simulink model "sampleModel106"  (R2022a)
settings: Solver=VariableStepAuto  StartTime=0.0  StopTime=10.0  RelTol=1e-3
undefined symbols (not defined in the file): DiscIntNeverNeededParam, magnitude, Newton, Raphson
libraries: simulink x379, slpidlib x89
(part 7 of 16)

== system sampleModel106/cfblk74/cfblk13/cfblk11/cfblk9 ==
  cfblk1 : Inport
  cfblk9 : Inport  Port=2
  cfblk10 : Inport  Port=3
  cfblk3 : slpidlib/PID Controller (2DOF)  Controller=PID  Form=Parallel  TimeDomain=Discrete-time  UseExternalTs=off  SampleTime=1  IntegratorMethod=Forward Euler  FilterMethod=Forward Euler  ControllerParametersSource=internal  P=1  I=1  UseKiTs=off  D=0  N=100  UseFilter=on  b=1  c=1  TunerSelectOption=Transfer Function Based (PID Tuner App)  InitialConditionSource=internal  InitialConditionForIntegrator=0  InitialConditionForFilter=0  DifferentiatorICPrevScaledInput=0  ExternalReset=none  TrackingMode=off  Kt=1  LimitOutput=off  SatLimitsSource=internal  UpperSaturationLimit=inf  LowerSaturationLimit=-inf  LinearizeAsGain=off  AntiWindupMode=none  Kb=1  POutMin=[]  POutMax=[]  IOutMin=[]  IOutMax=[]  DOutMin=[]  DOutMax=[]  NOutMin=[]  NOutMax=[]  bOutMin=[]  bOutMax=[]  cOutMin=[]  cOutMax=[]  SumOutMin=[]  SumOutMax=[]  SaturationOutMin=[]  SaturationOutMax=[]  PParamMin=[]  PParamMax=[]  IParamMin=[]  IParamMax=[]  DParamMin=[]  DParamMax=[]  NParamMin=[]  NParamMax=[]  bParamMin=[]  bParamMax=[]  cParamMin=[]  cParamMax=[]  KbParamMin=[]  KbParamMax=[]  KtParamMin=[]  KtParamMax=[]  KbOutMin=[]  KbOutMax=[]  KtOutMin=[]  KtOutMax=[]  IntegratorOutMin=[]  IntegratorOutMax=[]  FilterOutMin=[]  FilterOutMax=[]  SumI1OutMin=[]  SumI1OutMax=[]  SumI2OutMin=[]  SumI2OutMax=[]  SumI3OutMin=[]  SumI3OutMax=[]  SumI4OutMin=[]  SumI4OutMax=[]  SumDOutMin=[]  SumDOutMax=[]  Sum1OutMin=[]  Sum1OutMax=[]  Sum2OutMin=[]  Sum2OutMax=[]  Sum3OutMin=[]  Sum3OutMax=[]  DifferentiatorOutMin=[]  DifferentiatorOutMax=[]  FilterDiffOutCoefMin=[]  FilterDiffOutCoefMax=[]  ReciprocalOutMin=[]  ReciprocalOutMax=[]  SumDenOutMin=[]  SumDenOutMax=[]  SumNumOutMin=[]  SumNumOutMax=[]  DivideOutMin=[]  DivideOutMax=[]  UdiffTsProdOutMin=[]  UdiffTsProdOutMax=[]  NTsProdOutMin=[]  NTsProdOutMax=[]  UintegralTsProdOutMin=[]  UintegralTsProdOutMax=[]  UngainTsProdOutMin=[]  UngainTsProdOutMax=[]  IntegratorContinuousStateAttributes=''  IntegratorStateMustResolveToSignalObject=off  IntegratorRTWStateStorageClass=Auto  FilterContinuousStateAttributes=''  FilterStateMustResolveToSignalObject=off  FilterRTWStateStorageClass=Auto  ParallelPVariant=InternalParameters  IdealPVariant=Disabled  IVariant=InternalParameters  DVariant=InternalParameters  bVariant=InternalParameters  cVariant=InternalParameters  IntegratorVariant=Discrete  SatVariant=Disabled  AWVariant=Passthrough  PCopyVariant=Disabled  TRVariant=Disabled  FdbkBlocksVariant=Forward  IdealPFdbkVariant=Disabled  SatFdbkVariant=Disabled  DerivativeFilterVariant=ForwardEulerFilter  NVariant=InternalParameters  NCopyVariant=Disabled  FilterICVariant=InternalICsFilter  IntegratorICVariant=InternalICs  ExternalResetVariant=Disabled  TRSumVariant=Passthrough  SumFdbkVariant=Disabled  SumVariant=Sum_PID  TsampFilterVariant=InternalTs  TsampNgainVariant=Passthrough  TsampIntegralVariant=Passthrough  ExternalSaturationOutDataTypeStr=Inherit: Same as second input
      settings: SourceProductBaseCode=SL
  cfblk4 : simulink/Discrete/Difference  ICPrevInput=0.0  OutMin=[]  OutMax=[]  OutDataTypeStr=Inherit: Inherit via back propagation  OutDataType=fixdt(1, 16)  OutScaling=2^-10  DoSatur=off
  cfblk5 : Delay  SampleTime=1
  cfblk6 : Constant  Value=[-806684680.192649]  SampleTime=1
  cfblk7 : Constant  Value=[-623429069.453188]  SampleTime=1
  cfblk8 : Constant  Value=[-163983169.490583]  SampleTime=1
  cfblk2 : Outport
  cfblk11 : Outport  Port=2
  cfblk12 : Outport  Port=3
  wires:
  cfblk8/1 -> cfblk11/1
  cfblk6/1 -> cfblk2/1
  cfblk7/1 -> cfblk12/1
  cfblk10/1 -> cfblk5/1
  cfblk5/1 -> cfblk3/1
  cfblk9/1 -> cfblk3/2
  cfblk3/1 -> cfblk4/1

== system sampleModel106/cfblk74/cfblk13/cfblk12/cfblk10 ==
  cfblk1 : Inport
  cfblk8 : Inport  Port=2
  cfblk9 : Inport  Port=3
  cfblk3 : Delay  SampleTime=1
  cfblk4 : Sin  TimeSource=Use external signal  SampleTime=0
  cfblk5 : Sum  Inputs=+
  cfblk6 : simulink/Math Operations/MinMax Running Resettable  Function=min  vinit=0.0
  cfblk7 : Constant  Value=[-796301996.468178]  SampleTime=1
  cfblk2 : Outport
  cfblk10 : Outport  Port=2
  wires:
  cfblk5/1 -> cfblk4/1
  cfblk4/1 -> cfblk10/1
  cfblk8/1 -> cfblk6/1
  cfblk9/1 -> cfblk2/1
  cfblk3/1 -> cfblk5/1
  cfblk6/1 -> cfblk3/1
  cfblk7/1 -> cfblk6/2

== system sampleModel106/cfblk74/cfblk13/cfblk13/cfblk10 ==
  cfblk1 : Inport
  cfblk12 : Inport  Port=2
  cfblk13 : Inport  Port=3
  cfblk14 : Inport  Port=4
  cfblk15 : Inport  Port=5
  cfblk10 : ComplexToMagnitudeAngle
  cfblk11 : Constant  Value=[-793901753.508385]  SampleTime=1
  cfblk3 : simulink/Discrete/Transfer Fcn First Order  PoleZ=0.95  ICPrevOutput=0.0  DoSatur=off
  cfblk4 : MinMax  Inputs=3
  cfblk5 : Sum  Inputs=--
  cfblk6 : Rounding
  cfblk7 : UnaryMinus
  cfblk8 : Sqrt
  cfblk9 : Product
  cfblk2 : Outport
  cfblk16 : Outport  Port=2
  wires:
  cfblk7/1 -> cfblk5/1
  cfblk10/1 -> cfblk3/1
  cfblk10/2 -> cfblk7/1
  cfblk12/1 -> cfblk6/1
  cfblk6/1 -> cfblk10/1
  cfblk4/1 -> cfblk16/1
  cfblk11/1 -> cfblk5/2
  cfblk15/1 -> cfblk4/1
  cfblk3/1 -> cfblk8/1
  cfblk8/1 -> cfblk2/1
  cfblk5/1 -> cfblk9/1
  cfblk9/1 -> cfblk4/2
  cfblk14/1 -> cfblk4/3
  cfblk13/1 -> cfblk9/2

== system sampleModel106/cfblk74/cfblk13/cfblk13/cfblk11 ==
  cfblk1 : Inport
  cfblk3 : Product  Inputs=*
  cfblk4 : Sqrt
  cfblk5 : Bias  Bias=[715168761.956103]  SaturateOnIntegerOverflow=off
  cfblk6 : ComplexToMagnitudeAngle
  cfblk7 : Signum
  cfblk8 : Delay  SampleTime=1
  cfblk9 : Delay  SampleTime=1
  cfblk2 : Outport
  wires:
  cfblk1/1 -> cfblk2/1
  cfblk4/1 -> cfblk5/1
  cfblk3/1 -> cfblk7/1
  cfblk7/1 -> cfblk6/1
  cfblk6/1 -> cfblk8/1
  cfblk8/1 -> cfblk3/1
  cfblk5/1 -> cfblk9/1
  cfblk9/1 -> cfblk4/1

== system sampleModel106/cfblk74/cfblk13/cfblk13/cfblk12 ==
  cfblk1 : Inport
  cfblk10 : Constant  Value=[-475820294.361022]  SampleTime=1
  cfblk11 : Constant  Value=[-225279314.465098]  SampleTime=1
  cfblk3 : simulink/Discrete/Transfer Fcn Lead or Lag  PoleZ=0.95  ZeroZ=0.75  ICPrevOutput=0.0  ICPrevInput=0.0  DoSatur=off
      settings: SourceProductBaseCode=SL
  cfblk4 : Trigonometry
  cfblk5 : Sum  Inputs=|++
  cfblk6 : Squeeze
  cfblk7 : Reshape
  cfblk8 : Constant  Value=[-614077669.222538]  SampleTime=1
  cfblk9 : Constant  Value=[-535025394.973729]  SampleTime=1
  cfblk2 : Outport
  cfblk12 : Outport  Port=2
  wires:
  cfblk5/1 -> cfblk3/1
  cfblk11/1 -> cfblk12/1
  cfblk8/1 -> cfblk7/1
  cfblk4/1 -> cfblk2/1
  cfblk9/1 -> cfblk4/1
  cfblk3/1 -> cfblk6/1
  cfblk1/1 -> cfblk5/1
  cfblk7/1 -> cfblk5/2

== system sampleModel106/cfblk74/cfblk13/cfblk13/cfblk9 ==
  cfblk1 : Inport
  cfblk7 : Inport  Port=2
  cfblk3 : simulink/Discrete/Transfer Fcn Real Zero  ZeroZ=0.75  ICPrevInput=0.0  DoSatur=off
      settings: SourceProductBaseCode=SL
  cfblk4 : Reshape
  cfblk5 : Rounding
  cfblk6 : Constant  Value=[-810853108.486231]  SampleTime=1
  cfblk2 : Outport
  cfblk8 : Outport  Port=2
  wires:
  cfblk4/1 -> cfblk3/1
  cfblk1/1 -> cfblk2/1
  cfblk7/1 -> cfblk5/1
  cfblk6/1 -> cfblk4/1
  cfblk5/1 -> cfblk8/1

== system sampleModel106/cfblk74/cfblk9/cfblk11/cfblk8 ==
  cfblk1 : Inport
  cfblk9 : Inport  Port=2
  cfblk10 : Inport  Port=3
  cfblk3 : Delay  ShowEnablePort=on  SampleTime=1
      settings: InputPortMap=u0,e6
  cfblk4 : Sqrt  Operator=rSqrt  AlgorithmType=Newton-Raphson
  cfblk5 : simulink/Math Operations/MinMax Running Resettable  Function=min  vinit=0.0
  cfblk6 : Constant  Value=[-597140278.382424]  SampleTime=1
  cfblk7 : Constant  Value=[926673631.119186]  SampleTime=1
  cfblk8 : Constant  Value=[-242832753.012015]  SampleTime=1
  cfblk2 : Outport
  cfblk11 : Outport  Port=2
  wires:
  cfblk10/1 -> cfblk11/1
  cfblk4/1 -> cfblk3/1
  cfblk9/1 -> cfblk5/1
  cfblk5/1 -> cfblk2/1
  cfblk8/1 -> cfblk3/2
  cfblk6/1 -> cfblk5/2
  cfblk1/1 -> cfblk4/1

== system sampleModel106/cfblk74/cfblk9/cfblk11/cfblk9 ==
  cfblk1 : Inport
  cfblk8 : Inport  Port=2
  cfblk3 : Signum
  cfblk4 : Sum  Inputs=+-
  cfblk5 : PermuteDimensions
  cfblk6 : Product  Inputs=**
  cfblk7 : Constant  Value=[458452339.303576]  SampleTime=1
  cfblk2 : Outport
  cfblk9 : Outport  Port=2
  wires:
  cfblk5/1 -> cfblk6/1
  cfblk7/1 -> cfblk4/1
  cfblk3/1 -> cfblk6/2
  cfblk6/1 -> cfblk9/1
  cfblk8/1 -> cfblk4/2, cfblk5/1
  cfblk1/1 -> cfblk2/1
  cfblk4/1 -> cfblk3/1

== system sampleModel106/cfblk74/cfblk9/cfblk12/cfblk10 ==
  cfblk1 : Inport
  cfblk6 : Inport  Port=2
  cfblk7 : Inport  Port=3
  cfblk3 : slpidlib/PID Controller (2DOF)  Controller=PID  Form=Parallel  TimeDomain=Discrete-time  UseExternalTs=off  SampleTime=1  IntegratorMethod=Forward Euler  FilterMethod=Forward Euler  ControllerParametersSource=internal  P=1  I=1  UseKiTs=off  D=0  N=100  UseFilter=on  b=1  c=1  TunerSelectOption=Transfer Function Based (PID Tuner App)  InitialConditionSource=internal  InitialConditionForIntegrator=0  InitialConditionForFilter=0  DifferentiatorICPrevScaledInput=0  ExternalReset=none  TrackingMode=off  Kt=1  LimitOutput=off  SatLimitsSource=internal  UpperSaturationLimit=inf  LowerSaturationLimit=-inf  LinearizeAsGain=off  AntiWindupMode=none  Kb=1  POutMin=[]  POutMax=[]  IOutMin=[]  IOutMax=[]  DOutMin=[]  DOutMax=[]  NOutMin=[]  NOutMax=[]  bOutMin=[]  bOutMax=[]  cOutMin=[]  cOutMax=[]  SumOutMin=[]  SumOutMax=[]  SaturationOutMin=[]  SaturationOutMax=[]  PParamMin=[]  PParamMax=[]  IParamMin=[]  IParamMax=[]  DParamMin=[]  DParamMax=[]  NParamMin=[]  NParamMax=[]  bParamMin=[]  bParamMax=[]  cParamMin=[]  cParamMax=[]  KbParamMin=[]  KbParamMax=[]  KtParamMin=[]  KtParamMax=[]  KbOutMin=[]  KbOutMax=[]  KtOutMin=[]  KtOutMax=[]  IntegratorOutMin=[]  IntegratorOutMax=[]  FilterOutMin=[]  FilterOutMax=[]  SumI1OutMin=[]  SumI1OutMax=[]  SumI2OutMin=[]  SumI2OutMax=[]  SumI3OutMin=[]  SumI3OutMax=[]  SumI4OutMin=[]  SumI4OutMax=[]  SumDOutMin=[]  SumDOutMax=[]  Sum1OutMin=[]  Sum1OutMax=[]  Sum2OutMin=[]  Sum2OutMax=[]  Sum3OutMin=[]  Sum3OutMax=[]  DifferentiatorOutMin=[]  DifferentiatorOutMax=[]  FilterDiffOutCoefMin=[]  FilterDiffOutCoefMax=[]  ReciprocalOutMin=[]  ReciprocalOutMax=[]  SumDenOutMin=[]  SumDenOutMax=[]  SumNumOutMin=[]  SumNumOutMax=[]  DivideOutMin=[]  DivideOutMax=[]  UdiffTsProdOutMin=[]  UdiffTsProdOutMax=[]  NTsProdOutMin=[]  NTsProdOutMax=[]  UintegralTsProdOutMin=[]  UintegralTsProdOutMax=[]  UngainTsProdOutMin=[]  UngainTsProdOutMax=[]  IntegratorContinuousStateAttributes=''  IntegratorStateMustResolveToSignalObject=off  IntegratorRTWStateStorageClass=Auto  FilterContinuousStateAttributes=''  FilterStateMustResolveToSignalObject=off  FilterRTWStateStorageClass=Auto  ParallelPVariant=InternalParameters  IdealPVariant=Disabled  IVariant=InternalParameters  DVariant=InternalParameters  bVariant=InternalParameters  cVariant=InternalParameters  IntegratorVariant=Discrete  SatVariant=Disabled  AWVariant=Passthrough  PCopyVariant=Disabled  TRVariant=Disabled  FdbkBlocksVariant=Forward  IdealPFdbkVariant=Disabled  SatFdbkVariant=Disabled  DerivativeFilterVariant=ForwardEulerFilter  NVariant=InternalParameters  NCopyVariant=Disabled  FilterICVariant=InternalICsFilter  IntegratorICVariant=InternalICs  ExternalResetVariant=Disabled  TRSumVariant=Passthrough  SumFdbkVariant=Disabled  SumVariant=Sum_PID  TsampFilterVariant=InternalTs  TsampNgainVariant=Passthrough  TsampIntegralVariant=Passthrough  ExternalSaturationOutDataTypeStr=Inherit: Same as second input
      settings: SourceProductBaseCode=SL
  cfblk4 : DiscreteZeroPole  Poles=[0 0.5]  Gain=1
  cfblk5 : Gain  Gain=[955284268.719632]
  cfblk8 : Delay  SampleTime=1
  cfblk2 : Outport
  wires:
  cfblk5/1 -> cfblk4/1
  cfblk1/1 -> cfblk3/1
  cfblk3/1 -> cfblk5/1
  cfblk6/1 -> cfblk2/1
  cfblk4/1 -> cfblk8/1
  cfblk8/1 -> cfblk3/2

== system sampleModel106/cfblk74/cfblk9/cfblk12/cfblk13 ==
  cfblk1 : Inport
  cfblk12 : Inport  Port=2
  cfblk13 : Inport  Port=3
  Action Port : ActionPort  ActionPortLabel=if(u1 >= 0)
  cfblk10 : Constant  Value=[-679946503.878796]  SampleTime=1
  cfblk11 : Constant  Value=[-962530128.203573]  SampleTime=1
  cfblk17 : Delay
  cfblk3 : Sum
  cfblk4 : Sum  Inputs=+-
  cfblk5 : Trigonometry
  cfblk6 : Sum  Inputs=+-
  cfblk7 : Squeeze
  cfblk8 : Constant  Value=[916836463.739358]  SampleTime=1
  cfblk9 : Constant  Value=[-400818000.791556]  SampleTime=1
  cfblk2 : Outport
  cfblk14 : Outport  Port=2
  cfblk15 : Outport  Port=3
  cfblk16 : Outport  Port=4
  wires:
  cfblk3/1 -> cfblk4/1
  cfblk11/1 -> cfblk14/1
  cfblk5/1 -> cfblk2/1
  cfblk7/1 -> cfblk3/1
  cfblk9/1 -> cfblk15/1
  cfblk12/1 -> cfblk6/1
  cfblk6/1 -> cfblk4/2
  cfblk1/1 -> cfblk16/1
  cfblk8/1 -> cfblk7/1
  cfblk13/1 -> cfblk6/2
  cfblk10/1 -> cfblk5/1
  cfblk4/1 -> cfblk17/1
  cfblk17/1 -> cfblk3/2

== system sampleModel106/cfblk74/cfblk9/cfblk12/cfblk14 ==
  cfblk1 : Inport
  cfblk9 : Inport  Port=2
  cfblk10 : Inport  Port=3
  cfblk11 : Inport  Port=4
  Action Port : ActionPort  ActionPortLabel=else
  cfblk3 : DiscreteTransferFcn
  cfblk4 : Squeeze
  cfblk5 : Product
  cfblk6 : Constant  Value=[-850030709.629340]  SampleTime=1
  cfblk7 : Constant  Value=[320075082.603753]  SampleTime=1
  cfblk8 : Constant  Value=[416679782.582926]  SampleTime=1
  cfblk2 : Outport
  cfblk12 : Outport  Port=2
  wires:
  cfblk6/1 -> cfblk5/1
  cfblk11/1 -> cfblk4/1
  cfblk5/1 -> cfblk2/1
  cfblk4/1 -> cfblk3/1
  cfblk1/1 -> cfblk5/2
  cfblk3/1 -> cfblk12/1

== system sampleModel106/cfblk74/cfblk9/cfblk12/cfblk8 ==
  cfblk1 : Inport
  cfblk7 : Inport  Port=2
  cfblk3 : PermuteDimensions
  cfblk4 : simulink/Math Operations/Slider Gain  gain=1  low=0  high=2
  cfblk5 : Gain  Gain=[356985907.848455]
  cfblk6 : Sum  Inputs=+-
  cfblk8 : Delay  SampleTime=1
  cfblk2 : Outport
  wires:
  cfblk7/1 -> cfblk2/1, cfblk5/1
  cfblk6/1 -> cfblk4/1
  cfblk1/1 -> cfblk3/1
  cfblk3/1 -> cfblk6/2
  cfblk4/1 -> cfblk8/1
  cfblk8/1 -> cfblk6/1

== system sampleModel106/cfblk74/cfblk9/cfblk12/cfblk9 ==
  cfblk1 : Inport
  cfblk8 : Inport  Port=2
  cfblk9 : Inport  Port=3
  cfblk10 : Inport  Port=4
  cfblk3 : simulink/Discrete/Transfer Fcn Lead or Lag  PoleZ=0.95  ZeroZ=0.75  ICPrevOutput=0.0  ICPrevInput=0.0  DoSatur=off
      settings: SourceProductBaseCode=SL
  cfblk4 : ComplexToMagnitudeAngle
  cfblk5 : Rounding
  cfblk6 : Sum  Inputs=-+
  cfblk7 : Gain  Gain=[630253926.006221]
  cfblk2 : Outport
  wires:
  cfblk6/1 -> cfblk5/1
  cfblk3/1 -> cfblk7/1
  cfblk10/1 -> cfblk6/1
  cfblk5/1 -> cfblk4/1
  cfblk1/1 -> cfblk6/2
  cfblk8/1 -> cfblk2/1
  cfblk9/1 -> cfblk3/1

== system sampleModel106/cfblk74/cfblk9/cfblk13/cfblk5 ==
  cfblk1 : Inport
  cfblk9 : Inport  Port=2
  cfblk3 : DiscreteFir  SampleTime=1
  cfblk4 : DiscreteIntegrator  ICPrevOutput=DiscIntNeverNeededParam  ICPrevScaledInput=DiscIntNeverNeededParam
  cfblk5 : slpidlib/PID Controller  Controller=PID  Form=Parallel  TimeDomain=Discrete-time  UseExternalTs=off  SampleTime=1  IntegratorMethod=Forward Euler  FilterMethod=Forward Euler  ControllerParametersSource=internal  P=1  I=1  UseKiTs=off  D=0  N=100  UseFilter=on  TunerSelectOption=Transfer Function Based (PID Tuner App)  InitialConditionSource=internal  InitialConditionForIntegrator=0  InitialConditionForFilter=0  DifferentiatorICPrevScaledInput=0  ExternalReset=none  TrackingMode=off  Kt=1  LimitOutput=off  SatLimitsSource=internal  UpperSaturationLimit=inf  LowerSaturationLimit=-inf  LinearizeAsGain=off  AntiWindupMode=none  Kb=1  POutMin=[]  POutMax=[]  IOutMin=[]  IOutMax=[]  DOutMin=[]  DOutMax=[]  NOutMin=[]  NOutMax=[]  SumOutMin=[]  SumOutMax=[]  SaturationOutMin=[]  SaturationOutMax=[]  PParamMin=[]  PParamMax=[]  IParamMin=[]  IParamMax=[]  DParamMin=[]  DParamMax=[]  NParamMin=[]  NParamMax=[]  KbParamMin=[]  KbParamMax=[]  KtParamMin=[]  KtParamMax=[]  KbOutMin=[]  KbOutMax=[]  KtOutMin=[]  KtOutMax=[]  IntegratorOutMin=[]  IntegratorOutMax=[]  FilterOutMin=[]  FilterOutMax=[]  SumI1OutMin=[]  SumI1OutMax=[]  SumI2OutMin=[]  SumI2OutMax=[]  SumI3OutMin=[]  SumI3OutMax=[]  SumI4OutMin=[]  SumI4OutMax=[]  SumDOutMin=[]  SumDOutMax=[]  DifferentiatorOutMin=[]  DifferentiatorOutMax=[]  FilterDiffOutCoefMin=[]  FilterDiffOutCoefMax=[]  ReciprocalOutMin=[]  ReciprocalOutMax=[]  SumDenOutMin=[]  SumDenOutMax=[]  SumNumOutMin=[]  SumNumOutMax=[]  DivideOutMin=[]  DivideOutMax=[]  UdiffTsProdOutMin=[]  UdiffTsProdOutMax=[]  NTsProdOutMin=[]  NTsProdOutMax=[]  UintegralTsProdOutMin=[]  UintegralTsProdOutMax=[]  UngainTsProdOutMin=[]  UngainTsProdOutMax=[]  IntegratorContinuousStateAttributes=''  IntegratorStateMustResolveToSignalObject=off  IntegratorRTWStateStorageClass=Auto  FilterContinuousStateAttributes=''  FilterStateMustResolveToSignalObject=off  FilterRTWStateStorageClass=Auto  ParallelPVariant=InternalParameters  IdealPVariant=Disabled  IVariant=InternalParameters  DVariant=InternalParameters  IntegratorVariant=Discrete  SatVariant=Disabled  AWVariant=Passthrough  PCopyVariant=Disabled  TRVariant=Disabled  FdbkBlocksVariant=Forward  IdealPFdbkVariant=Disabled  SatFdbkVariant=Disabled  DerivativeFilterVariant=ForwardEulerFilter  NVariant=InternalParameters  NCopyVariant=Disabled  FilterICVariant=InternalICsFilter  IntegratorICVariant=InternalICs  ExternalResetVariant=Disabled  TRSumVariant=Passthrough  SumFdbkVariant=Disabled  SumVariant=Sum_PID  TsampFilterVariant=InternalTs  TsampNgainVariant=Passthrough  TsampIntegralVariant=Passthrough  ExternalSaturationOutDataTypeStr=Inherit: Same as second input  aMode=0
  cfblk6 : MinMax
  cfblk7 : Gain  Gain=[65666299.408699]
  cfblk8 : Constant  Value=[554029224.863969]  SampleTime=1
  cfblk2 : Outport
  cfblk10 : Outport  Port=2
  wires:
  cfblk6/1 -> cfblk5/1
  cfblk8/1 -> cfblk7/1
  cfblk9/1 -> cfblk10/1
  cfblk7/1 -> cfblk6/1
  cfblk5/1 -> cfblk3/1
  cfblk3/1 -> cfblk4/1
  cfblk1/1 -> cfblk2/1

== system sampleModel106/cfblk74/cfblk9/cfblk13/cfblk6 ==
  cfblk1 : Inport
  cfblk7 : Inport  Port=2
  cfblk8 : Inport  Port=3
  cfblk10 : Delay  SampleTime=1
  cfblk3 : DiscreteTransferFcn  SampleTime=1
  cfblk4 : UnitDelay  HasFrameUpgradeWarning=on
  cfblk5 : DiscreteIntegrator  ICPrevOutput=DiscIntNeverNeededParam  ICPrevScaledInput=DiscIntNeverNeededParam
  cfblk6 : UnaryMinus
  cfblk2 : Outport
  cfblk9 : Outport  Port=2
  wires:
  cfblk5/1 -> cfblk2/1
  cfblk3/1 -> cfblk4/1
  cfblk1/1 -> cfblk9/1
  cfblk4/1 -> cfblk6/1
  cfblk7/1 -> cfblk5/1
  cfblk6/1 -> cfblk10/1
  cfblk10/1 -> cfblk3/1

== system sampleModel106/cfblk74/cfblk9/cfblk13/cfblk7 ==
  cfblk1 : Inport
  cfblk10 : Sqrt
  cfblk11 : Constant  Value=[49726155.340751]  SampleTime=1
  cfblk12 : Constant  Value=[51502285.530327]  SampleTime=1
  cfblk14 : Delay  SampleTime=1
  cfblk3 : simulink/Discrete/Transfer Fcn Lead or Lag  PoleZ=0.95  ZeroZ=0.75  ICPrevOutput=0.0  ICPrevInput=0.0  DoSatur=off
      settings: SourceProductBaseCode=SL
  cfblk4 : Sum  Inputs=+-
  cfblk5 : Trigonometry
  cfblk6 : simulink/Math Operations/Slider Gain  gain=1  low=0  high=2
  cfblk7 : MinMax  Function=max  Inputs=2
  cfblk8 : Sqrt
  cfblk9 : Math  Operator=10^u
  cfblk2 : Outport
  cfblk13 : Outport  Port=2
  wires:
  cfblk1/1 -> cfblk5/1
  cfblk12/1 -> cfblk3/1
  cfblk4/1 -> cfblk8/1
  cfblk9/1 -> cfblk6/1
  cfblk3/1 -> cfblk9/1, cfblk4/2
  cfblk6/1 -> cfblk2/1
  cfblk8/1 -> cfblk10/1
  cfblk5/1 -> cfblk7/1
  cfblk11/1 -> cfblk7/2
  cfblk7/1 -> cfblk13/1
  cfblk10/1 -> cfblk14/1
  cfblk14/1 -> cfblk4/1

== system sampleModel106/cfblk74/cfblk9/cfblk15/cfblk10 ==
  cfblk1 : Inport
  cfblk11 : Inport  Port=2
  cfblk10 : Constant  Value=[231958979.755721]  SampleTime=1
  cfblk3 : DiscreteFilter  SampleTime=1
  cfblk4 : Product  Inputs=*
  cfblk5 : Gain  Gain=[-64902621.159940]
  cfblk6 : Reshape
  cfblk7 : Sum  Inputs=+
  cfblk8 : Constant  Value=[-549811752.008296]  SampleTime=1
  cfblk9 : Constant  Value=[666189529.416412]  SampleTime=1
  cfblk2 : Outport
  cfblk12 : Outport  Port=2
  wires:
  cfblk9/1 -> cfblk6/1
  cfblk1/1 -> cfblk3/1
  cfblk6/1 -> cfblk5/1
  cfblk10/1 -> cfblk7/1
  cfblk5/1 -> cfblk2/1
  cfblk11/1 -> cfblk4/1
  cfblk3/1 -> cfblk12/1

== system sampleModel106/cfblk74/cfblk9/cfblk15/cfblk11 ==
  cfblk1 : Inport
  cfblk13 : Inport  Port=2
  cfblk14 : Inport  Port=3
  cfblk10 : Constant  Value=[-458676472.570737]  SampleTime=1
  cfblk11 : Constant  Value=[-707014969.582165]  SampleTime=1
  cfblk12 : Constant  Value=[815086080.140174]  SampleTime=1
  cfblk17 : Delay  SampleTime=1
  cfblk3 : slpidlib/PID Controller (2DOF)  Controller=PID  Form=Parallel  TimeDomain=Discrete-time  UseExternalTs=off  SampleTime=1  IntegratorMethod=Forward Euler  FilterMethod=Forward Euler  ControllerParametersSource=internal  P=1  I=1  UseKiTs=off  D=0  N=100  UseFilter=on  b=1  c=1  TunerSelectOption=Transfer Function Based (PID Tuner App)  InitialConditionSource=internal  InitialConditionForIntegrator=0  InitialConditionForFilter=0  DifferentiatorICPrevScaledInput=0  ExternalReset=none  TrackingMode=off  Kt=1  LimitOutput=off  SatLimitsSource=internal  UpperSaturationLimit=inf  LowerSaturationLimit=-inf  LinearizeAsGain=off  AntiWindupMode=none  Kb=1  POutMin=[]  POutMax=[]  IOutMin=[]  IOutMax=[]  DOutMin=[]  DOutMax=[]  NOutMin=[]  NOutMax=[]  bOutMin=[]  bOutMax=[]  cOutMin=[]  cOutMax=[]  SumOutMin=[]  SumOutMax=[]  SaturationOutMin=[]  SaturationOutMax=[]  PParamMin=[]  PParamMax=[]  IParamMin=[]  IParamMax=[]  DParamMin=[]  DParamMax=[]  NParamMin=[]  NParamMax=[]  bParamMin=[]  bParamMax=[]  cParamMin=[]  cParamMax=[]  KbParamMin=[]  KbParamMax=[]  KtParamMin=[]  KtParamMax=[]  KbOutMin=[]  KbOutMax=[]  KtOutMin=[]  KtOutMax=[]  IntegratorOutMin=[]  IntegratorOutMax=[]  FilterOutMin=[]  FilterOutMax=[]  SumI1OutMin=[]  SumI1OutMax=[]  SumI2OutMin=[]  SumI2OutMax=[]  SumI3OutMin=[]  SumI3OutMax=[]  SumI4OutMin=[]  SumI4OutMax=[]  SumDOutMin=[]  SumDOutMax=[]  Sum1OutMin=[]  Sum1OutMax=[]  Sum2OutMin=[]  Sum2OutMax=[]  Sum3OutMin=[]  Sum3OutMax=[]  DifferentiatorOutMin=[]  DifferentiatorOutMax=[]  FilterDiffOutCoefMin=[]  FilterDiffOutCoefMax=[]  ReciprocalOutMin=[]  ReciprocalOutMax=[]  SumDenOutMin=[]  SumDenOutMax=[]  SumNumOutMin=[]  SumNumOutMax=[]  DivideOutMin=[]  DivideOutMax=[]  UdiffTsProdOutMin=[]  UdiffTsProdOutMax=[]  NTsProdOutMin=[]  NTsProdOutMax=[]  UintegralTsProdOutMin=[]  UintegralTsProdOutMax=[]  UngainTsProdOutMin=[]  UngainTsProdOutMax=[]  IntegratorContinuousStateAttributes=''  IntegratorStateMustResolveToSignalObject=off  IntegratorRTWStateStorageClass=Auto  FilterContinuousStateAttributes=''  FilterStateMustResolveToSignalObject=off  FilterRTWStateStorageClass=Auto  ParallelPVariant=InternalParameters  IdealPVariant=Disabled  IVariant=InternalParameters  DVariant=InternalParameters  bVariant=InternalParameters  cVariant=InternalParameters  IntegratorVariant=Discrete  SatVariant=Disabled  AWVariant=Passthrough  PCopyVariant=Disabled  TRVariant=Disabled  FdbkBlocksVariant=Forward  IdealPFdbkVariant=Disabled  SatFdbkVariant=Disabled  DerivativeFilterVariant=ForwardEulerFilter  NVariant=InternalParameters  NCopyVariant=Disabled  FilterICVariant=InternalICsFilter  IntegratorICVariant=InternalICs  ExternalResetVariant=Disabled  TRSumVariant=Passthrough  SumFdbkVariant=Disabled  SumVariant=Sum_PID  TsampFilterVariant=InternalTs  TsampNgainVariant=Passthrough  TsampIntegralVariant=Passthrough  ExternalSaturationOutDataTypeStr=Inherit: Same as second input
      settings: SourceProductBaseCode=SL
  cfblk4 : DiscreteTransferFcn  SampleTime=1
  cfblk5 : Delay  SampleTime=1
  cfblk6 : DiscreteIntegrator  ICPrevOutput=DiscIntNeverNeededParam  ICPrevScaledInput=DiscIntNeverNeededParam
  cfblk7 : Reshape
  cfblk8 : Squeeze
  cfblk9 : Constant  Value=[869825865.592683]  SampleTime=1
  cfblk2 : Outport
  cfblk15 : Outport  Port=2
  cfblk16 : Outport  Port=3
  wires:
  cfblk9/1 -> cfblk2/1
  cfblk10/1 -> cfblk6/1
  cfblk7/1 -> cfblk8/1
  cfblk5/1 -> cfblk16/1
  cfblk3/1 -> cfblk7/1
  cfblk13/1 -> cfblk5/1
  cfblk12/1 -> cfblk15/1
  cfblk1/1 -> cfblk4/1
  cfblk6/1 -> cfblk3/2
  cfblk8/1 -> cfblk17/1
  cfblk17/1 -> cfblk3/1

== system sampleModel106/cfblk74/cfblk9/cfblk15/cfblk9 ==
  cfblk1 : Inport
  cfblk7 : Inport  Port=2
  cfblk8 : Inport  Port=3
  cfblk3 : Delay  DelayLengthSource=Input port  SampleTime=1
      settings: InputPortMap=u0,p1
  cfblk4 : simulink/Discrete/Difference  ICPrevInput=0.0  OutMin=[]  OutMax=[]  OutDataTypeStr=Inherit: Inherit via back propagation  OutDataType=fixdt(1, 16)  OutScaling=2^-10  DoSatur=off
  cfblk5 : Product  Inputs=**
  cfblk6 : Constant  Value=[-105116644.466995]  SampleTime=1
  cfblk9 : Delay  SampleTime=1
  cfblk2 : Outport
  wires:
  cfblk6/1 -> cfblk3/1
  cfblk1/1 -> cfblk2/1
  cfblk4/1 -> cfblk5/1
  cfblk3/1 -> cfblk4/1
  cfblk8/1 -> cfblk5/2
  cfblk5/1 -> cfblk9/1
  cfblk9/1 -> cfblk3/2

== system sampleModel106/cfblk74/cfblk9/cfblk16/cfblk7 ==
  cfblk1 : Inport
  cfblk7 : Inport  Port=2
  cfblk8 : Inport  Port=3
  cfblk3 : simulink/Discrete/Difference  ICPrevInput=0.0  OutMin=[]  OutMax=[]  OutDataTypeStr=Inherit: Inherit via back propagation  OutDataType=fixdt(1, 16)  OutScaling=2^-10  DoSatur=off
  cfblk4 : ComplexToRealImag
  cfblk5 : Sum  Inputs=+-
  cfblk6 : Constant  Value=[101423658.427814]  SampleTime=1
  cfblk2 : Outport
  wires:
  cfblk4/1 -> cfblk5/1
  cfblk8/1 -> cfblk2/1
  cfblk7/1 -> cfblk4/1
  cfblk6/1 -> cfblk3/1
  cfblk3/1 -> cfblk5/2

== system sampleModel106/cfblk74/cfblk9/cfblk16/cfblk8 ==
  cfblk1 : Inport
  cfblk14 : Inport  Port=2
  cfblk15 : Inport  Port=3
  cfblk10 : Squeeze
  cfblk11 : Reshape
  cfblk12 : simulink/Math Operations/Slider Gain  gain=1  low=0  high=2
  cfblk13 : Constant  Value=[-734947851.856283]  SampleTime=1
  cfblk17 : Delay  SampleTime=1
  cfblk18 : Delay  SampleTime=1
  cfblk3 : Delay  ShowEnablePort=on  SampleTime=1
      settings: InputPortMap=u0,e6
  cfblk4 : Delay  SampleTime=1
  cfblk5 : DiscreteFilter  SampleTime=1
  cfblk6 : simulink/Discrete/Difference  ICPrevInput=0.0  OutMin=[]  OutMax=[]  OutDataTypeStr=Inherit: Inherit via back propagation  OutDataType=fixdt(1, 16)  OutScaling=2^-10  DoSatur=off
  cfblk7 : Trigonometry
  cfblk8 : MinMax  Function=max
  cfblk9 : Trigonometry
  cfblk2 : Outport
  cfblk16 : Outport  Port=2
  wires:
  cfblk12/1 -> cfblk10/1
  cfblk10/1 -> cfblk6/1
  cfblk14/1 -> cfblk2/1
  cfblk7/1 -> cfblk9/1
  cfblk15/1 -> cfblk16/1
  cfblk1/1 -> cfblk12/1
  cfblk11/1 -> cfblk8/1
  cfblk3/1 -> cfblk11/1
  cfblk13/1 -> cfblk4/1
  cfblk5/1 -> cfblk7/1
  cfblk6/1 -> cfblk3/1
  cfblk8/1 -> cfblk17/1
  cfblk17/1 -> cfblk3/2
  cfblk9/1 -> cfblk18/1
  cfblk18/1 -> cfblk5/1

== system sampleModel106/cfblk74/cfblk9/cfblk9/cfblk10 ==
  cfblk1 : Inport
  cfblk10 : Inport  Port=2
  cfblk11 : Inport  Port=3
  cfblk12 : Inport  Port=4
  cfblk13 : Delay  SampleTime=1
  cfblk3 : Delay  ShowEnablePort=on  SampleTime=1
      settings: InputPortMap=u0,e6
  cfblk4 : DiscreteStateSpace
  cfblk5 : Rounding
  cfblk6 : Abs  SaturateOnIntegerOverflow=off
  cfblk7 : Product  Inputs=*
  cfblk8 : Sum  Inputs=+-
  cfblk9 : Constant  Value=[839535444.416101]  SampleTime=1
  cfblk2 : Outport
  wires:
  cfblk3/1 -> cfblk4/1
  cfblk4/1 -> cfblk2/1
  cfblk11/1 -> cfblk8/1
  cfblk5/1 -> cfblk7/1
  cfblk9/1 -> cfblk3/1
  cfblk1/1 -> cfblk8/2
  cfblk12/1 -> cfblk6/1
  cfblk10/1 -> cfblk3/2
  cfblk7/1 -> cfblk13/1
  cfblk13/1 -> cfblk5/1

== system sampleModel106/cfblk74/cfblk9/cfblk9/cfblk11 ==
  cfblk1 : Inport
  cfblk6 : Inport  Port=2
  cfblk7 : Inport  Port=3
  cfblk8 : Inport  Port=4
  cfblk3 : Delay  ShowEnablePort=on  SampleTime=1
      settings: InputPortMap=u0,e6
  cfblk4 : simulink/Discrete/Transfer Fcn Lead or Lag  PoleZ=0.95  ZeroZ=0.75  ICPrevOutput=0.0  ICPrevInput=0.0  DoSatur=off
      settings: SourceProductBaseCode=SL
  cfblk5 : Sum  Inputs=|++
  cfblk9 : Delay  SampleTime=1
  cfblk2 : Outport
  wires:
  cfblk7/1 -> cfblk2/1
  cfblk1/1 -> cfblk3/1
  cfblk4/1 -> cfblk5/1
  cfblk6/1 -> cfblk3/2
  cfblk8/1 -> cfblk5/2
  cfblk5/1 -> cfblk9/1
  cfblk9/1 -> cfblk4/1

== system sampleModel106/cfblk74/cfblk9/cfblk9/cfblk9 ==
  cfblk1 : Inport
  cfblk10 : Constant  Value=[-213956286.197865]  SampleTime=1
  cfblk12 : Delay  SampleTime=1
  cfblk3 : DiscreteIntegrator  ICPrevOutput=DiscIntNeverNeededParam  ICPrevScaledInput=DiscIntNeverNeededParam
  cfblk4 : simulink/Math Operations/Slider Gain  gain=1  low=0  high=2
  cfblk5 : Gain  Gain=[-650980414.519220]
  cfblk6 : Sum
  cfblk7 : Bias  Bias=[254600432.308890]  SaturateOnIntegerOverflow=off
  cfblk8 : Sum
  cfblk9 : Constant  Value=[-488733431.313732]  SampleTime=1
  cfblk2 : Outport
  cfblk11 : Outport  Port=2
  wires:
  cfblk4/1 -> cfblk8/1
  cfblk9/1 -> cfblk11/1
  cfblk6/1 -> cfblk5/1
  cfblk5/1 -> cfblk2/1, cfblk12/1
  cfblk8/1 -> cfblk6/2
  cfblk10/1 -> cfblk3/1
  cfblk1/1 -> cfblk7/1
  cfblk3/1 -> cfblk8/2
  cfblk7/1 -> cfblk4/1
  cfblk12/1 -> cfblk6/1

== system sampleModel106/cfblk75/cfblk5/cfblk10/cfblk10 ==
  cfblk1 : Inport
  cfblk7 : Inport  Port=2
  Action Port : ActionPort  ActionPortLabel=if(u1 >= 0)
  cfblk3 : DiscreteFir
  cfblk4 : Sqrt  Operator=rSqrt  AlgorithmType=Newton-Raphson
  cfblk5 : ComplexToRealImag
  cfblk6 : Constant  Value=[-367349926.183283]  SampleTime=1
  cfblk2 : Outport
  wires:
  cfblk7/1 -> cfblk3/1
  cfblk1/1 -> cfblk5/1
  cfblk3/1 -> cfblk4/1
  cfblk4/1 -> cfblk2/1

== system sampleModel106/cfblk75/cfblk5/cfblk10/cfblk11 ==
  cfblk1 : Inport
  cfblk6 : Inport  Port=2
  cfblk7 : Inport  Port=3
  Action Port : ActionPort  ActionPortLabel=else
  cfblk3 : simulink/Discrete/Difference  ICPrevInput=0.0  OutMin=[]  OutMax=[]  OutDataTypeStr=Inherit: Inherit via back propagation  OutDataType=fixdt(1, 16)  OutScaling=2^-10  DoSatur=off
  cfblk4 : Rounding
  cfblk5 : UnaryMinus
  cfblk2 : Outport
  wires:
  cfblk1/1 -> cfblk4/1
  cfblk7/1 -> cfblk3/1
  cfblk6/1 -> cfblk5/1
  cfblk3/1 -> cfblk2/1

== system sampleModel106/cfblk75/cfblk5/cfblk10/cfblk7 ==
  cfblk1 : Inport
  cfblk8 : Inport  Port=2
  cfblk9 : Inport  Port=3
  cfblk3 : Delay  SampleTime=1
  cfblk4 : Constant  Value=[153261747.093953]  SampleTime=1
  cfblk5 : Constant  Value=[301665033.109607]  SampleTime=1
  cfblk6 : Constant  Value=[495999944.454875]  SampleTime=1
  cfblk7 : Constant  Value=[-896329617.684975]  SampleTime=1
  cfblk2 : Outport
  cfblk10 : Outport  Port=2
  wires:
  cfblk1/1 -> cfblk3/1
  cfblk4/1 -> cfblk2/1
  cfblk6/1 -> cfblk10/1

== system sampleModel106/cfblk75/cfblk5/cfblk10/cfblk8 ==
  cfblk1 : Inport
  cfblk9 : Inport  Port=2
  cfblk3 : simulink/Discrete/Transfer Fcn First Order  PoleZ=0.95  ICPrevOutput=0.0  DoSatur=off
  cfblk4 : Delay  SampleTime=1
  cfblk5 : Abs  SaturateOnIntegerOverflow=off
  cfblk6 : Sum  Inputs=+
  cfblk7 : Constant  Value=[-421735980.173699]  SampleTime=1
  cfblk8 : Constant  Value=[-284767442.051453]  SampleTime=1
  cfblk2 : Outport
  wires:
  cfblk4/1 -> cfblk5/1
  cfblk1/1 -> cfblk4/1
  cfblk5/1 -> cfblk3/1
  cfblk7/1 -> cfblk6/1
  cfblk6/1 -> cfblk2/1

== system sampleModel106/cfblk75/cfblk5/cfblk11/cfblk10 ==
  cfblk1 : Inport
  cfblk9 : Inport  Port=2
  cfblk10 : Inport  Port=3
  cfblk3 : slpidlib/PID Controller (2DOF)  Controller=PID  Form=Parallel  TimeDomain=Discrete-time  UseExternalTs=off  SampleTime=1  IntegratorMethod=Forward Euler  FilterMethod=Forward Euler  ControllerParametersSource=internal  P=1  I=1  UseKiTs=off  D=0  N=100  UseFilter=on  b=1  c=1  TunerSelectOption=Transfer Function Based (PID Tuner App)  InitialConditionSource=internal  InitialConditionForIntegrator=0  InitialConditionForFilter=0  DifferentiatorICPrevScaledInput=0  ExternalReset=none  TrackingMode=off  Kt=1  LimitOutput=off  SatLimitsSource=internal  UpperSaturationLimit=inf  LowerSaturationLimit=-inf  LinearizeAsGain=off  AntiWindupMode=none  Kb=1  POutMin=[]  POutMax=[]  IOutMin=[]  IOutMax=[]  DOutMin=[]  DOutMax=[]  NOutMin=[]  NOutMax=[]  bOutMin=[]  bOutMax=[]  cOutMin=[]  cOutMax=[]  SumOutMin=[]  SumOutMax=[]  SaturationOutMin=[]  SaturationOutMax=[]  PParamMin=[]  PParamMax=[]  IParamMin=[]  IParamMax=[]  DParamMin=[]  DParamMax=[]  NParamMin=[]  NParamMax=[]  bParamMin=[]  bParamMax=[]  cParamMin=[]  cParamMax=[]  KbParamMin=[]  KbParamMax=[]  KtParamMin=[]  KtParamMax=[]  KbOutMin=[]  KbOutMax=[]  KtOutMin=[]  KtOutMax=[]  IntegratorOutMin=[]  IntegratorOutMax=[]  FilterOutMin=[]  FilterOutMax=[]  SumI1OutMin=[]  SumI1OutMax=[]  SumI2OutMin=[]  SumI2OutMax=[]  SumI3OutMin=[]  SumI3OutMax=[]  SumI4OutMin=[]  SumI4OutMax=[]  SumDOutMin=[]  SumDOutMax=[]  Sum1OutMin=[]  Sum1OutMax=[]  Sum2OutMin=[]  Sum2OutMax=[]  Sum3OutMin=[]  Sum3OutMax=[]  DifferentiatorOutMin=[]  DifferentiatorOutMax=[]  FilterDiffOutCoefMin=[]  FilterDiffOutCoefMax=[]  ReciprocalOutMin=[]  ReciprocalOutMax=[]  SumDenOutMin=[]  SumDenOutMax=[]  SumNumOutMin=[]  SumNumOutMax=[]  DivideOutMin=[]  DivideOutMax=[]  UdiffTsProdOutMin=[]  UdiffTsProdOutMax=[]  NTsProdOutMin=[]  NTsProdOutMax=[]  UintegralTsProdOutMin=[]  UintegralTsProdOutMax=[]  UngainTsProdOutMin=[]  UngainTsProdOutMax=[]  IntegratorContinuousStateAttributes=''  IntegratorStateMustResolveToSignalObject=off  IntegratorRTWStateStorageClass=Auto  FilterContinuousStateAttributes=''  FilterStateMustResolveToSignalObject=off  FilterRTWStateStorageClass=Auto  ParallelPVariant=InternalParameters  IdealPVariant=Disabled  IVariant=InternalParameters  DVariant=InternalParameters  bVariant=InternalParameters  cVariant=InternalParameters  IntegratorVariant=Discrete  SatVariant=Disabled  AWVariant=Passthrough  PCopyVariant=Disabled  TRVariant=Disabled  FdbkBlocksVariant=Forward  IdealPFdbkVariant=Disabled  SatFdbkVariant=Disabled  DerivativeFilterVariant=ForwardEulerFilter  NVariant=InternalParameters  NCopyVariant=Disabled  FilterICVariant=InternalICsFilter  IntegratorICVariant=InternalICs  ExternalResetVariant=Disabled  TRSumVariant=Passthrough  SumFdbkVariant=Disabled  SumVariant=Sum_PID  TsampFilterVariant=InternalTs  TsampNgainVariant=Passthrough  TsampIntegralVariant=Passthrough  ExternalSaturationOutDataTypeStr=Inherit: Same as second input
      settings: SourceProductBaseCode=SL
  cfblk4 : MinMax  Inputs=3
  cfblk5 : Sqrt  Operator=rSqrt  AlgorithmType=Newton-Raphson
  cfblk6 : Assignment  DiagnosticForDimensions=Warning  IndexOptions=Index vector (dialog)  Indices=1  OutputSizes=1
  cfblk7 : Constant  Value=[-373145141.474232]  SampleTime=1
  cfblk8 : Constant  Value=[56367090.496888]  SampleTime=1
  cfblk2 : Outport
  cfblk11 : Outport  Port=2
  wires:
  cfblk6/1 -> cfblk11/1
  cfblk7/1 -> cfblk5/1
  cfblk10/1 -> cfblk4/1
  cfblk9/1 -> cfblk3/1
  cfblk4/1 -> cfblk3/2
  cfblk5/1 -> cfblk2/1, cfblk4/3
  cfblk1/1 -> cfblk6/1
  cfblk8/1 -> cfblk4/2
  cfblk3/1 -> cfblk6/2

== system sampleModel106/cfblk75/cfblk5/cfblk9/cfblk10 ==
  cfblk1 : Inport
  cfblk14 : Inport  Port=2
  cfblk15 : Inport  Port=3
  cfblk10 : Product
  cfblk11 : Sqrt  Operator=rSqrt  AlgorithmType=Newton-Raphson
  cfblk12 : Constant  Value=[-873906557.460500]  SampleTime=1
  cfblk13 : Constant  Value=[-37663214.804296]  SampleTime=1
  cfblk3 : UnitDelay  HasFrameUpgradeWarning=on
  cfblk4 : simulink/Discrete/Difference  ICPrevInput=0.0  OutMin=[]  OutMax=[]  OutDataTypeStr=Inherit: Inherit via back propagation  OutDataType=fixdt(1, 16)  OutScaling=2^-10  DoSatur=off
  cfblk5 : UnitDelay  HasFrameUpgradeWarning=on
  cfblk6 : ComplexToRealImag
  cfblk7 : Bias  Bias=[260361926.921988]  SaturateOnIntegerOverflow=off
  cfblk8 : Sqrt  Operator=rSqrt  AlgorithmType=Newton-Raphson
  cfblk9 : Product
  cfblk2 : Outport
  wires:
  cfblk1/1 -> cfblk10/1
  cfblk8/1 -> cfblk4/1
  cfblk14/1 -> cfblk11/1
  cfblk11/1 -> cfblk9/1
  cfblk10/1 -> cfblk2/1
  cfblk7/1 -> cfblk9/2
  cfblk6/1 -> cfblk3/1
  cfblk4/1 -> cfblk7/1
  cfblk5/1 -> cfblk6/1
  cfblk15/1 -> cfblk8/1
  cfblk13/1 -> cfblk5/1
  cfblk9/1 -> cfblk10/2

== system sampleModel106/cfblk75/cfblk5/cfblk9/cfblk8 ==
  cfblk1 : Inport
  cfblk8 : Inport  Port=2
  cfblk9 : Inport  Port=3
  cfblk3 : simulink/Discrete/Tapped Delay  vinit=0.0  samptime=-1  NumDelays=1  DelayOrder=Oldest  includeCurrent=off
  cfblk4 : Sqrt
  cfblk5 : Product  Inputs=**
  cfblk6 : Product  Inputs=**
  cfblk7 : Constant  Value=[484093966.380805]  SampleTime=1
  cfblk2 : Outport
  wires:
  cfblk9/1 -> cfblk4/1
  cfblk7/1 -> cfblk3/1
  cfblk5/1 -> cfblk2/1
  cfblk6/1 -> cfblk5/1
  cfblk4/1 -> cfblk5/2
  cfblk3/1 -> cfblk6/1
  cfblk1/1 -> cfblk6/2

== system sampleModel106/cfblk75/cfblk5/cfblk9/cfblk9 ==
  cfblk1 : Inport
  cfblk16 : Inport  Port=2
  cfblk10 : DotProduct  OutDataTypeStr=Inherit: Inherit via internal rule
  cfblk11 : Gain  Gain=[-188661269.583772]
  cfblk12 : simulink/Math Operations/Slider Gain  gain=1  low=0  high=2
  cfblk13 : Gain  Gain=[-202396196.825646]
  cfblk14 : Trigonometry
  cfblk15 : Sum  Inputs=+-
  cfblk17 : Delay  SampleTime=1
  cfblk18 : Delay  SampleTime=1
  cfblk19 : Delay  SampleTime=1
  cfblk3 : UnitDelay  HasFrameUpgradeWarning=on
  cfblk4 : DiscreteStateSpace
  cfblk5 : simulink/Discrete/Transfer Fcn Lead or Lag  PoleZ=0.95  ZeroZ=0.75  ICPrevOutput=0.0  ICPrevInput=0.0  DoSatur=off
      settings: SourceProductBaseCode=SL
  cfblk6 : simulink/Discrete/Transfer Fcn Lead or Lag  PoleZ=0.95  ZeroZ=0.75  ICPrevOutput=0.0  ICPrevInput=0.0  DoSatur=off
      settings: SourceProductBaseCode=SL
  cfblk7 : DiscreteFir  SampleTime=1
  cfblk8 : Bias  Bias=[877229886.360265]  SaturateOnIntegerOverflow=off
  cfblk9 : Polyval  Coefs=[ +2.081618890e-019, -1.441693666e-014, +4.719686976e-010, -8.536869453e-006, +1.621573104e-001, -8.087801117e+001 ]
  cfblk2 : Outport
  wires:
  cfblk5/1 -> cfblk7/1, cfblk6/1
  cfblk4/1 -> cfblk12/1
  cfblk14/1 -> cfblk13/1
  cfblk9/1 -> cfblk2/1
  cfblk7/1 -> cfblk11/1
  cfblk12/1 -> cfblk8/1
  cfblk10/1 -> cfblk4/1
  cfblk3/1 -> cfblk14/1
  cfblk11/1 -> cfblk9/1
  cfblk1/1 -> cfblk15/1
  cfblk15/1 -> cfblk10/2
  cfblk16/1 -> cfblk15/2
  cfblk8/1 -> cfblk17/1
  cfblk17/1 -> cfblk10/1
  cfblk13/1 -> cfblk18/1
  cfblk18/1 -> cfblk3/1
  cfblk6/1 -> cfblk19/1
  cfblk19/1 -> cfblk5/1

== system sampleModel106/cfblk75/cfblk6/cfblk5/cfblk7 ==
  cfblk1 : Inport
  cfblk9 : Inport  Port=2
  cfblk3 : UnaryMinus
  cfblk4 : Signum
  cfblk5 : Constant  Value=[407618625.499441]  SampleTime=1
  cfblk6 : Constant  Value=[812064205.889443]  SampleTime=1
  cfblk7 : Constant  Value=[542609041.875015]  SampleTime=1
  cfblk8 : Constant  Value=[390772971.886045]  SampleTime=1
  cfblk2 : Outport
  cfblk10 : Outport  Port=2
  wires:
  cfblk8/1 -> cfblk10/1
  cfblk9/1 -> cfblk2/1
  cfblk4/1 -> cfblk3/1
  cfblk7/1 -> cfblk4/1

== system sampleModel106/cfblk75/cfblk6/cfblk6/cfblk13 ==
  cfblk1 : Inport
  cfblk9 : Inport  Port=2
  cfblk10 : Delay  SampleTime=1
  cfblk11 : Delay  SampleTime=1
  cfblk3 : Delay  DelayLengthSource=Input port  SampleTime=1
      settings: InputPortMap=u0,p1
  cfblk4 : Sum  Inputs=+
  cfblk5 : Sum  Inputs=--
  cfblk6 : Sum  Inputs=+-
  cfblk7 : PermuteDimensions
  cfblk8 : Sqrt  Operator=rSqrt  AlgorithmType=Newton-Raphson
  cfblk2 : Outport
  wires:
  cfblk1/1 -> cfblk5/1
  cfblk5/1 -> cfblk3/1
  cfblk7/1 -> cfblk10/1, cfblk11/1
  cfblk6/1 -> cfblk7/1
  cfblk9/1 -> cfblk4/1, cfblk8/1
  cfblk8/1 -> cfblk2/1
  cfblk3/1 -> cfblk6/2
  cfblk4/1 -> cfblk3/2
  cfblk10/1 -> cfblk6/1
  cfblk11/1 -> cfblk5/2

== system sampleModel106/cfblk75/cfblk6/cfblk6/cfblk14 ==
  cfblk1 : Inport
  cfblk12 : Inport  Port=2
  cfblk13 : Inport  Port=3
  cfblk10 : Constant  Value=[-832645924.853920]  SampleTime=1
  cfblk11 : Constant  Value=[-288956008.710308]  SampleTime=1
  cfblk15 : Delay  SampleTime=1
  cfblk3 : simulink/Discrete/Transfer Fcn Lead or Lag  PoleZ=0.95  ZeroZ=0.75  ICPrevOutput=0.0  ICPrevInput=0.0  DoSatur=off
      settings: SourceProductBaseCode=SL
  cfblk4 : DiscreteFilter  SampleTime=1
  cfblk5 : Sin  TimeSource=Use external signal  SampleTime=0
  cfblk6 : ComplexToRealImag
  cfblk7 : Bias  Bias=[-793808167.408014]  SaturateOnIntegerOverflow=off
  cfblk8 : Math  Operator=hypot
  cfblk9 : Product
  cfblk2 : Outport
  cfblk14 : Outport  Port=2
  wires:
  cfblk1/1 -> cfblk2/1
  cfblk10/1 -> cfblk5/1
  cfblk4/1 -> cfblk9/1
  cfblk11/1 -> cfblk9/2
  cfblk8/1 -> cfblk4/1
  cfblk7/1 -> cfblk8/2
  cfblk6/1 -> cfblk3/1
  cfblk3/1 -> cfblk7/1
  cfblk13/1 -> cfblk14/1
  cfblk12/1 -> cfblk6/1
  cfblk9/1 -> cfblk15/1
  cfblk15/1 -> cfblk8/1

== system sampleModel106/cfblk75/cfblk6/cfblk7/cfblk9 ==
  cfblk1 : Inport
  cfblk8 : Inport  Port=2
  cfblk9 : Inport  Port=3
  cfblk10 : Inport  Port=4
  cfblk3 : Sqrt  Operator=rSqrt  AlgorithmType=Newton-Raphson
  cfblk4 : UnaryMinus
  cfblk5 : Sin  TimeSource=Use external signal  SampleTime=0
  cfblk6 : Abs  SaturateOnIntegerOverflow=off
  cfblk7 : Constant  Value=[715822373.797498]  SampleTime=1
  cfblk2 : Outport
  wires:
  cfblk3/1 -> cfblk5/1
  cfblk7/1 -> cfblk2/1
  cfblk9/1 -> cfblk4/1
  cfblk6/1 -> cfblk3/1
  cfblk8/1 -> cfblk6/1

== system sampleModel106/cfblk75/cfblk6/cfblk8/cfblk10 ==
  cfblk1 : Inport
  cfblk10 : Inport  Port=2
  cfblk11 : Inport  Port=3
  cfblk12 : Inport  Port=4
  cfblk3 : DiscreteFir  SampleTime=1
  cfblk4 : simulink/Math Operations/Slider Gain  gain=1  low=0  high=2
  cfblk5 : Signum
  cfblk6 : Sqrt
  cfblk7 : simulink/Math Operations/MinMax Running Resettable  Function=min  vinit=0.0
  cfblk8 : Constant  Value=[-630356113.466739]  SampleTime=1
  cfblk9 : Constant  Value=[714306692.800453]  SampleTime=1
  cfblk2 : Outport
  wires:
  cfblk5/1 -> cfblk3/1
  cfblk6/1 -> cfblk7/1
  cfblk11/1 -> cfblk4/1
  cfblk1/1 -> cfblk2/1
  cfblk7/1 -> cfblk5/1
  cfblk9/1 -> cfblk7/2
  cfblk10/1 -> cfblk6/1

== system sampleModel106/cfblk75/cfblk6/cfblk8/cfblk11 ==
  cfblk1 : Inport
  cfblk10 : Inport  Port=2
  cfblk{3..4,12..13} (4 alike) : Delay  SampleTime=1
  cfblk5 : Delay  ShowEnablePort=on  SampleTime=1
      settings: InputPortMap=u0,e6
  cfblk6 : PermuteDimensions
  cfblk7 : Signum
  cfblk8 : Sum  Inputs=+
  cfblk9 : Sum  Inputs=+
  cfblk2 : Outport
  cfblk11 : Outport  Port=2
  wires:
  cfblk6/1 -> cfblk3/1
  cfblk7/1 -> cfblk6/1
  cfblk9/1 -> cfblk12/1, cfblk13/1
  cfblk1/1 -> cfblk8/1
  cfblk8/1 -> cfblk2/1
  cfblk4/1 -> cfblk11/1
  cfblk5/1 -> cfblk9/1
  cfblk10/1 -> cfblk7/1
  cfblk3/1 -> cfblk4/1
  cfblk12/1 -> cfblk5/1
  cfblk13/1 -> cfblk5/2

== system sampleModel106/cfblk75/cfblk6/cfblk8/cfblk12 ==
  cfblk1 : Inport
  cfblk8 : Inport  Port=2
  cfblk3 : simulink/Discrete/Transfer Fcn Real Zero  ZeroZ=0.75  ICPrevInput=0.0  DoSatur=off
      settings: SourceProductBaseCode=SL
  cfblk4 : Sin  TimeSource=Use external signal  SampleTime=0
  cfblk5 : simulink/Math Operations/Slider Gain  gain=1  low=0  high=2
  cfblk6 : Sum  Inputs=+
  cfblk7 : Constant  Value=[-693080125.642337]  SampleTime=1
  cfblk2 : Outport
  wires:
  cfblk7/1 -> cfblk5/1
  cfblk5/1 -> cfblk6/1
  cfblk6/1 -> cfblk2/1
  cfblk4/1 -> cfblk3/1
  cfblk8/1 -> cfblk4/1

== system sampleModel106/cfblk75/cfblk6/cfblk8/cfblk9 ==
  cfblk1 : Inport
  cfblk11 : Inport  Port=2
  cfblk12 : Inport  Port=3
  cfblk10 : Constant  Value=[-242342768.401582]  SampleTime=1
  cfblk3 : simulink/Discrete/Transfer Fcn Real Zero  ZeroZ=0.75  ICPrevInput=0.0  DoSatur=off
      settings: SourceProductBaseCode=SL
  cfblk4 : simulink/Discrete/Transfer Fcn Real Zero  ZeroZ=0.75  ICPrevInput=0.0  DoSatur=off
      settings: SourceProductBaseCode=SL
  cfblk5 : UnaryMinus
  cfblk6 : PermuteDimensions
  cfblk7 : Polyval  Coefs=[ +2.081618890e-019, -1.441693666e-014, +4.719686976e-010, -8.536869453e-006, +1.621573104e-001, -8.087801117e+001 ]
  cfblk8 : Constant  Value=[340296221.064588]  SampleTime=1
  cfblk9 : Constant  Value=[-294608499.533957]  SampleTime=1
  cfblk2 : Outport
  cfblk13 : Outport  Port=2
  cfblk14 : Outport  Port=3
  cfblk15 : Outport  Port=4
  wires:
  cfblk10/1 -> cfblk6/1
  cfblk5/1 -> cfblk7/1
  cfblk8/1 -> cfblk5/1
  cfblk12/1 -> cfblk4/1
  cfblk7/1 -> cfblk2/1
  cfblk3/1 -> cfblk14/1
  cfblk11/1 -> cfblk13/1
  cfblk4/1 -> cfblk15/1
  cfblk6/1 -> cfblk3/1

== system sampleModel106/cfblk75/cfblk7/cfblk13/cfblk15 ==
  cfblk1 : Inport
  cfblk6 : Inport  Port=2
  cfblk7 : Inport  Port=3
  cfblk8 : Inport  Port=4
  cfblk9 : Inport  Port=5
  cfblk10 : Inport  Port=6
  cfblk11 : Inport  Port=7
  Action Port : ActionPort  ActionPortLabel=if(u1 >= 0)
  cfblk3 : Product
  cfblk4 : Sin  TimeSource=Use external signal  SampleTime=0
  cfblk5 : Constant  Value=[-300459830.684997]  SampleTime=1
  cfblk2 : Outport
  cfblk12 : Outport  Port=2
  cfblk13 : Outport  Port=3
  wires:
  cfblk7/1 -> cfblk3/1
  cfblk3/1 -> cfblk12/1
  cfblk9/1 -> cfblk13/1
  cfblk10/1 -> cfblk4/1
  cfblk6/1 -> cfblk3/2
  cfblk5/1 -> cfblk2/1

== system sampleModel106/cfblk75/cfblk7/cfblk13/cfblk16 ==
  cfblk1 : Inport
  cfblk12 : Inport  Port=2
  cfblk13 : Inport  Port=3
  Action Port : ActionPort  ActionPortLabel=else
  cfblk10 : Constant  Value=[274032633.093474]  SampleTime=1
  cfblk11 : Constant  Value=[-762082971.588581]  SampleTime=1
  cfblk3 : DiscreteFir
  cfblk4 : MinMax  Function=max
  cfblk5 : Abs  SaturateOnIntegerOverflow=off
  cfblk6 : Signum
  cfblk7 : PermuteDimensions
  cfblk8 : Product  Inputs=**
  cfblk9 : Trigonometry
  cfblk2 : Outport
  cfblk14 : Outport  Port=2
  cfblk15 : Outport  Port=3
  cfblk16 : Outport  Port=4
  wires:
  cfblk6/1 -> cfblk9/1
  cfblk4/1 -> cfblk5/1
  cfblk7/1 -> cfblk8/1
  cfblk12/1 -> cfblk3/1
  cfblk11/1 -> cfblk7/1
  cfblk3/1 -> cfblk15/1
  cfblk8/1 -> cfblk14/1
  cfblk9/1 -> cfblk2/1
  cfblk10/1 -> cfblk4/1
  cfblk1/1 -> cfblk8/2
  cfblk5/1 -> cfblk6/1
  cfblk13/1 -> cfblk16/1

== system sampleModel106/cfblk75/cfblk7/cfblk13/cfblk5 ==
  cfblk1 : Inport
  cfblk11 : Inport  Port=2
  cfblk12 : Inport  Port=3
  cfblk10 : Constant  Value=[-813416728.823410]  SampleTime=1
  cfblk16 : Delay
  cfblk3 : Signum
  cfblk4 : DotProduct  OutDataTypeStr=Inherit: Inherit via internal rule
  cfblk5 : Sqrt
  cfblk6 : Assignment  DiagnosticForDimensions=Warning  IndexOptions=Index vector (dialog)  Indices=1  OutputSizes=1
  cfblk7 : Product
  cfblk8 : Gain  Gain=[632096772.141171]
  cfblk9 : Constant  Value=[972939698.696570]  SampleTime=1
  cfblk2 : Outport
  cfblk13 : Outport  Port=2
  cfblk14 : Outport  Port=3
  cfblk15 : Outport  Port=4
  wires:
  cfblk12/1 -> cfblk3/1
  cfblk8/1 -> cfblk5/1
  cfblk9/1 -> cfblk4/1
  cfblk1/1 -> cfblk15/1
  cfblk11/1 -> cfblk8/1, cfblk6/2
  cfblk10/1 -> cfblk7/1
  cfblk4/1 -> cfblk7/2
  cfblk3/1 -> cfblk14/1
  cfblk5/1 -> cfblk6/1
  cfblk6/1 -> cfblk13/1, cfblk2/1
  cfblk7/1 -> cfblk16/1
  cfblk16/1 -> cfblk4/2

== system sampleModel106/cfblk75/cfblk7/cfblk13/cfblk6 ==
  cfblk1 : Inport
  cfblk8 : Inport  Port=2
  cfblk9 : Inport  Port=3
  cfblk10 : Inport  Port=4
  cfblk11 : Inport  Port=5
  cfblk3 : simulink/Discrete/Transfer Fcn First Order  PoleZ=0.95  ICPrevOutput=0.0  DoSatur=off
  cfblk4 : Bias  Bias=[-310481187.547714]  SaturateOnIntegerOverflow=off
  cfblk5 : Sin  TimeSource=Use external signal  SampleTime=0
  cfblk6 : simulink/Math Operations/Slider Gain  gain=1  low=0  high=2
  cfblk7 : Constant  Value=[41646868.952031]  SampleTime=1
  cfblk2 : Outport
  wires:
  cfblk6/1 -> cfblk4/1
  cfblk5/1 -> cfblk3/1
  cfblk11/1 -> cfblk5/1
  cfblk9/1 -> cfblk6/1
  cfblk1/1 -> cfblk2/1

== system sampleModel106/cfblk75/cfblk7/cfblk13/cfblk7 ==
  cfblk1 : Inport
  cfblk9 : Inport  Port=2
  cfblk10 : Inport  Port=3
  cfblk3 : ComplexToMagnitudeAngle
  cfblk4 : Signum
  cfblk5 : Constant  Value=[-714264542.321805]  SampleTime=1
  cfblk6 : Constant  Value=[-540741202.979561]  SampleTime=1
  cfblk7 : Constant  Value=[100464627.200416]  SampleTime=1
  cfblk8 : Constant  Value=[447981577.434649]  SampleTime=1
  cfblk2 : Outport
  cfblk11 : Outport  Port=2
  cfblk12 : Outport  Port=3
  wires:
  cfblk5/1 -> cfblk3/1
  cfblk10/1 -> cfblk2/1
  cfblk6/1 -> cfblk11/1
  cfblk4/1 -> cfblk12/1
  cfblk3/1 -> cfblk4/1

== system sampleModel106/cfblk75/cfblk7/cfblk13/cfblk8 ==
  cfblk1 : Inport
  cfblk9 : Inport  Port=2
  cfblk10 : Inport  Port=3
  cfblk12 : Delay
  cfblk3 : DiscreteZeroPole  Poles=[0 0.5]  Gain=1  SampleTime=-1
  cfblk4 : Sqrt  Operator=rSqrt  AlgorithmType=Newton-Raphson
  cfblk5 : Trigonometry
  cfblk6 : Sum  Inputs=+-
  cfblk7 : Polyval  Coefs=[ +2.081618890e-019, -1.441693666e-014, +4.719686976e-010, -8.536869453e-006, +1.621573104e-001, -8.087801117e+001 ]
  cfblk8 : Constant  Value=[-344560351.720051]  SampleTime=1
  cfblk2 : Outport
  cfblk11 : Outport  Port=2
  wires:
  cfblk3/1 -> cfblk4/1
  cfblk6/1 -> cfblk5/1
  cfblk10/1 -> cfblk11/1
  cfblk5/1 -> cfblk2/1
  cfblk8/1 -> cfblk6/1
  cfblk9/1 -> cfblk6/2
  cfblk1/1 -> cfblk7/1
  cfblk4/1 -> cfblk12/1
  cfblk12/1 -> cfblk3/1
